simulink model "SIMULINK_PID_ADP_Tracking_R18b - 副本"  (R2018b)
settings: Solver=FixedStepAuto  StartTime=0.0  StopTime=sim_end_time  FixedStep=fixed_step_size  RelTol=1e-3
InitFcn:
  | start_uav_car_10
undefined symbols (not defined in the file): a, act_end, b, battery_threshold, bb, delta_, draw_gif, droneyeeUAV2_NUM, droneyeeUAV3_NUM, droneyeeUAV4_NUM, droneyeeUAV5_NUM, fixed_step_size, k, KD_x, KD_y, kd_z, KDD_x, KDD_y, KI_x, KI_y, ki_z, KII_x, KII_y, KP_x, KP_y, kp_z, KPP_x, KPP_y, lmt, omega, omega_, R, sim_end_time, uav10num, uav1num, uav2num, uav3num, uav4num, uav5num, uav6num, uav7num, uav8num, uav9num, UAV_NUM, Vel_Switch_1, Vel_Switch_10, Vel_Switch_11, Vel_Switch_12, Vel_Switch_13, Vel_Switch_14, Vel_Switch_15, Vel_Switch_16, Vel_Switch_17, Vel_Switch_18, Vel_Switch_19, Vel_Switch_2, Vel_Switch_20, Vel_Switch_3, Vel_Switch_4, Vel_Switch_5 ... (+16)
libraries: simulink x121, aerolibanimutils x1
(part 11 of 11)

== matlab function SIMULINK_PID_ADP_Tracking_R18b - 副本/control system_UAV/Baseline Controller3/Position controller/X-Y ADP tracking controller/Obstacle detection ==
  data: X input; y output; Cache1 output
function [y,Cache1] = LCOA(X)
P_wp1=[10;30];  % target location

% x = X(1:2)-P_wp1;
x = X(1:2);
ro = 0.2;
ra = ro * 1.5;
rd = ro * 2;
L1 = 0.3; L2 = 0.8; L3 = 0.2;

% zk_ = [10 18; 18 18]-[P_wp1';P_wp1'];
% zk_ = [9-0.5 15; 17-0.5 15];
% zk_ = [9-1 15; 17-1 15];
% zk_ = [9-2 15; 17-2 15];
% zk_ = [1 15; 9 15];
% zk_ = [1.5 15; 8.5 15];
% zk_ = [2 15; 8 15];
% zk_ = [3 12; 7 18];
% zk_ = [3+0.5 15; 9 15];
% zk_ = [9 10; 11.5 25];
% zk_ = [10.5 15; 11.5 25];
zk_ = [-1.8 -0.6; -0.8 0.5];

s = 0; ds = [0;0];
beta = 0; dbeta = [0;0];

for i = 1:length(zk_)
    zk = zk_(i,:)';
    dk = norm(x-zk);
    ddk = (x-zk)/dk;
    betak = dk - ro;
    dbetak = ddk;
    
    if dk > rd
        sk = 0;
        dsk = [0;0];
    elseif dk >ra
        sk = L1 + L1 * cos(pi*(dk^2 - ra^2)/(rd^2 - ra^2));
        dsk = -2*pi*dk*ddk*sin(pi*(dk^2 - ra^2)/(rd^2 - ra^2))/(rd^2 - ra^2);
    elseif dk > ro
        sk = L2 + L3 * cos(pi*(dk^2 - ro^2)/(ra^2 - ro^2));
        dsk = -2*pi*dk*ddk*sin(pi*(dk^2 - ro^2)/(ra^2 - ro^2))/(ra^2 - ro^2);
    else
        sk = 1;
        dsk = [0;0];
    end
    ds = ds + dsk; s = s + sk;
    dbeta = dbeta + dbetak;
    beta = beta + betak;
end

mu = 0.01;
Kb = 5;
% Kb = 20;
% y = Kb * (dsk *(betak + mu) - dbetak * sk)/(betak + mu)^2; 
y = Kb * (ds *(beta + mu) - dbeta * s)/(beta + mu)^2; 


P_wp1=[10;30];  % target location

rrr=[ro;ra;rd];
Cache1=[rrr;P_wp1;zk_(1,:)';zk_(2,:)']; % input for plot111.m

== matlab function SIMULINK_PID_ADP_Tracking_R18b - 副本/control system_UAV/Baseline Controller3/Position controller/X-Y ADP tracking controller/adp_tracking ==
  data: P_feedback1 input; ux1 output; p_virtual1 input; Joystick input; delta_his input; omega_his input; W input; t input; dP_feedback1 input; lcoa input; uy1 output; delta_ output; omega_ output; dW_ output; test output
function [ux1,uy1,delta_,omega_,dW_,test] = adp_tracking(P_feedback1,p_virtual1,Joystick,delta_his,omega_his,W,t,dP_feedback1,lcoa)
% the parameter of 'approaching'

% P_wp1=[10;30];  % target location

sampleTime = 1/25;
g = 9.8;
A = zeros(2);
B = eye(2)/g;
% B = [zeros(2);eye(2)]/g;
Q = 100*eye(2);
R = 200*eye(2);
% R = 500*eye(2);

l = length(W);

dx = dP_feedback1;
% dx = u;

%% ADP Path Planning

% x = P_feedback1 - P_wp1;
x = P_feedback1 - p_virtual1;
x1 = x(1); x2 = x(2);
% phi = [x1^2;x1*x2;x2^2];
% dphi = [2*x1 0; x2 x1; 0 2*x2];
[sig,sig_p] = Staf_Basis(x); % State-following NN basis
dphi = sig_p;
test = norm(dphi);


%% update
% W = 1*[30.7119   42.8391  115.4889]';
umax = 1;
u_adp = -umax*tanh(0.5/umax*R\B'*dphi'*W);
% u_adp = -0.5*R\B'*dphi'*W;
u_safe = -0.5*R\B*lcoa;
u_adp = u_adp + u_safe;% + u_human;
% u_adp = -0.5*R\B'*dphi'*W;
% u_adp = lambda * u_adp + (1-lambda) * u_safe;
% K_lqr = [0.7071 0.0000; 0.0000 0.7071]*2;
% u_adp = -K_lqr*x;

if t > 10
%     u = u_adp;
%     u = -0.5*R\B'*dphi'*W;
    u = -umax*tanh(0.5/umax*R\B'*dphi'*W);
else
    u = zeros(2,1);
end
%% ADP nn

omega = dphi*dx;
delta = W'*omega + x'*Q*x + u'*R*u;
rou = 1 + omega'*omega;
delta_ = [delta_his(2:end,:); delta];
omega_ = [omega_his(2:end,:); omega'];

%% Concurrent learning
con_flag = 0;
if con_flag == 1 && t>10
    temp = zeros(l,1);
    for i = 1:length(delta_his)
        omega = omega_(i,:);
        delta = delta_(i,:);
        rou = 1 + omega*omega';
        temp = temp - 0.01*omega'./rou^2*delta; 
    end
    dW_ = temp;
elseif t>10
        dW_ = - 1*omega*delta/rou; 
else
        dW_ = zeros(l,1);
end
%% 输出
% u_adp = u;
ux1 = u_adp(1);
uy1 = u_adp(2);

== matlab function SIMULINK_PID_ADP_Tracking_R18b - 副本/control system_UAV/Baseline Controller3/Position controller/X-Y ADP tracking controller/reference_traj ==
  data: t input; p_ref input; dp_ref output; u_adp output
function [dp_ref,u_adp] = reference_traj(t,p_ref)
g = 9.8;
A = zeros(2);
B = eye(2)/g;
Q = 10*eye(2);
% R = 10*eye(2);
R = 100*eye(2);

P_wp1=[10;30];  % target location
x = p_ref - P_wp1;
x1 = x(1); x2 = x(2);

phi = [x1^2;x1*x2;x2^2];
dphi = [2*x1 0; x2 x1; 0 2*x2];
% [sig,sig_p] = Staf_Basis(x); % State-following NN basis
% dphi = sig_p;
umax = 15;

% W = [69.6962  194.1919  732.3164]';
% W = [240.3627  511.9875  480.4859]';
% W = [626.9039  661.0018  523.60190]';
W = [161.9089  606.9426  710.8552]';
% u_adp = -0.5*R\B'*dphi'*W;
if t > 12
    u_adp = -umax*tanh(0.5/umax*R\B'*dphi'*W);
else
    u_adp = zeros(2,1);
end
dp_ref = A*p_ref + B*u_adp;
